simulink model "geometric_controller_with_estimator"  (R2024b)
settings: Solver=VariableStepAuto  StartTime=0.0  StopTime=t(end)  RelTol=1e-3
InitFcn:
  | %% UAV PARAMETERS
  | m = 0.5;
  | Ib = diag([0.0023 0.0023 0.00509]);
  | %% UAV PARAMETERS
  | m = 0.5;
  | Ib = diag([0.0023 0.0023 0.00509]);
  | 
  | %% SAMPLING TIME
  | Ts=0.001;
  | 
  | %% TRAJECTORY
  | 
  | % time
  | t = t_tot;
  | 
  | % initial position
  | p0x = points(1,1);
  | p0y = points(1,2);
  | p0z = - points(1,3); % ENU -> NED
  | p0 = [p0x p0y p0z];
  | 
  | % trajectory
  | csi_d=p; dot_csi_d=p_dot; ddot_csi_d=p_ddot;
  | psi_d=zeros(1,length(t)); dot_psi_d=zeros(1,length(t)); ddot_psi_d=zeros(1,length(t));
values from neighbouring files (symbols this model uses):
  K = zeros(1,r)    [filter_coeff.m]
  p = [p segments(i:i+2,:)]    [main_trajectory.m]
  p_ddot = [p_ddot segments_ddot(i:i+2,:)]    [main_trajectory.m]
  p_dot = [p_dot segments_dot(i:i+2,:)]    [main_trajectory.m]
  points = zeros(n,3)    [casual_points.m]    (also in defined_points.m = [0 0 0.2)
  r = 1    [filter_coeff.m]
  t_tot = [t_tot t_temp(i,:)]    [main_trajectory.m]
undefined symbols (not defined in the file or in its folder): ceil_dim, ceil_p, DiscIntNeverNeededParam, par_dim, par_p, supp_dim, support_1_p, support_2_p
libraries: simulink x4, robotcorelib x3, dspsigops x2, uavutilslib x1
settings Model: Creator=fabioruggiero  LastModifiedBy=ricca
settings ModelReferenceCC: EnableRefExpFcnMdlSchedulingChecks=on
settings RTWCC: GPUComputeCapability=3.5

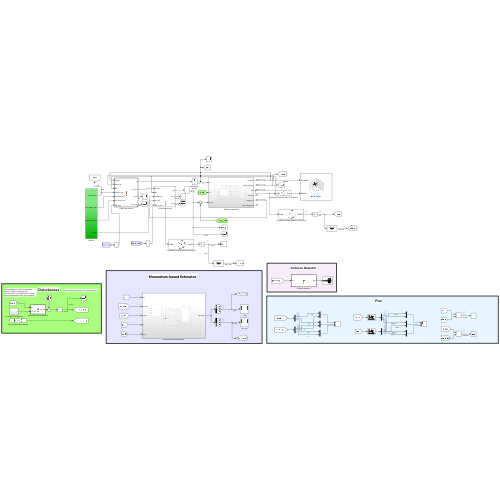
[thumbnail: Simulink's stored preview of the top-level diagram]
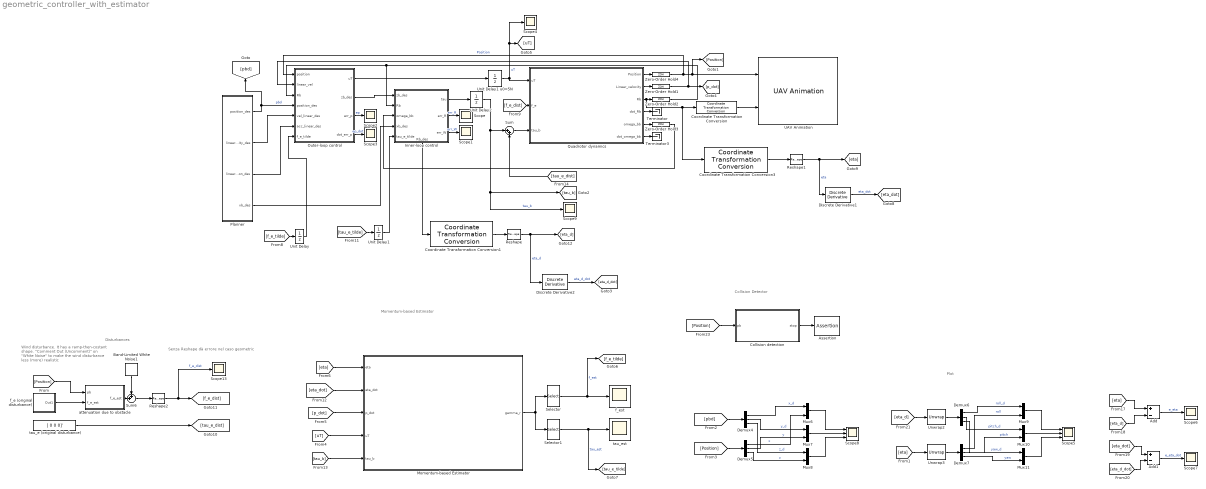
== system geometric_controller_with_estimator ==
  note: Momentum-based Estimator
  note: Collision Detector
  note: Plot
  note: Wind disturbance. It has a ramp-then-costant shape. "Comment Out (Uncomment)" on "White Noise" to make the wind disturbance less (more) realistic
  note: Senza Reshape dà errore nel caso geometric
  note: Disturbances
  Add : Sum  Inputs=+-
  Add1 : Sum  Inputs=+-
  Assertion : Assertion  AssertionFailFcn='WARNING: DRONE CRASHED!'
  Band-Limited White Noise1 : simulink/Sources/Band-Limited White Noise  Cov=[0.0001 0.0001 0]'  Ts=0.1  seed=[23341 23345 0]'  VectorParams1D=off
  Collision detection : MATLAB Function  TreatAsAtomicUnit=on
  Coordinate Transformation Conversion : robotcorelib/Coordinate Transformation Conversion  InputRepresentation=Rotation Matrix  InputEulerSequence=ZYX  ShowTrVecInputPort=on  OutputRepresentation=Quaternion  OutputEulerSequence=ZYX  ShowTrVecOutputPort=on  SimulateUsing=Interpreted execution
  Coordinate Transformation Conversion1 : robotcorelib/Coordinate Transformation Conversion  InputRepresentation=Rotation Matrix  InputEulerSequence=ZYX  ShowTrVecInputPort=on  OutputRepresentation=Euler Angles  OutputEulerSequence=XYZ  ShowTrVecOutputPort=on  SimulateUsing=Interpreted execution
  Coordinate Transformation Conversion3 : robotcorelib/Coordinate Transformation Conversion  InputRepresentation=Rotation Matrix  InputEulerSequence=ZYX  ShowTrVecInputPort=on  OutputRepresentation=Euler Angles  OutputEulerSequence=XYZ  ShowTrVecOutputPort=on  SimulateUsing=Interpreted execution
  Demux{4..7} (4 alike) : Demux  Outputs=3
  Discrete Derivative1 : simulink/Discrete/Discrete Derivative  gainval=1.0  ICPrevScaledInput=0.0  OutMin=[]  OutMax=[]  OutDataType=fixdt(1, 16)  OutScaling=2^-10  DoSatur=off
  Discrete Derivative2 : simulink/Discrete/Discrete Derivative  gainval=1.0  ICPrevScaledInput=0.0  OutMin=[]  OutMax=[]  OutDataType=fixdt(1, 16)  OutScaling=2^-10  DoSatur=off
  Inner-loop control : Subsystem  mask(Angular PID){Kr=10*eye(3), Kw=1*eye(3)}
      mask help: Kr, Kw ∈ R^(3x3) positive definite matrices
      settings: PortSchema="{\"entries\":[{\"content\":{\"sides\":[{\"content\":{\"connectorIds\":[\"In1\",\"In2\",\"In3\",\"In4\",\"In5\"]},\"type\":\"ConnectorPlacement.EquallySpacedRectSide\",\"uuid\":\"29c522b7-db36-4622-ad4a-717364e2cc35\"},{\"content\":{\"connectorIds\":[\"Out1\",\"Out2\",\"Out3\"],\"side\":\"RIGHT\"},\"type\":\"ConnectorPlacement.EquallySpacedRectSide\",\"uuid\":\"998238f4-a0c1-453d-a7e7-a110f68d17eb\"},{\"content\":{\"side\":\"TOP\"},\"type\":\"ConnectorPlacement.EquallySpacedRectSide\",\"uuid\":\"c0bfd343-7d48-415f-a23f-c8162a2dfc5d\"},{\"content\":{\"connectorIds\":[\"Out4\"],\"side\":\"BOTTOM\"},\"type\":\"ConnectorPlacement.EquallySpacedRectSide\",\"uuid\":\"eabcb074-d0a8-40eb-86b0-fc782e7c3bb4\"}]},\"type\":\"ConnectorPlacement.EquallySpacedConnector\",\"uuid\":\"fc5ab0de-d2d1-4caf-819d-5b1757328535\"}],\"packageUris\":[\"http://schema.mathworks.com/mf0/Connector/R2020b\"],\"version\":\"1.0\"}"
  Momentum-based Estimator : Subsystem
  Mux{6..11} (6 alike) : Mux  Inputs=2
  Outer-loop control : MATLAB Function  TreatAsAtomicUnit=on  mask(Linear PID){Kp=100*eye(3), Kv=100*eye(3)}
      mask help: Kp, Kv ∈ R^(3x3) positive definite matrices
  Planner : Subsystem
  Quadrotor dynamics : Subsystem
  Reshape : Reshape
  Reshape1 : Reshape
  Reshape2 : Reshape
  Scope{,1..4,6..7,9,13} (9 alike) : Scope
  Scope5 : Scope  NumInputPorts=3
  Scope8 : Scope  NumInputPorts=3
  Selector : Selector  InputPortWidth=6  IndexOptions=Index vector (dialog)  Indices=[1 2 3]  OutputSizes=1
  Selector1 : Selector  InputPortWidth=6  IndexOptions=Index vector (dialog)  Indices=[4 5 6]  OutputSizes=1
  Sum : Sum  Inputs=|++
  Sum6 : Sum  Inputs=++|
  Terminator : Terminator
  Terminator3 : Terminator
  UAV Animation : uavutilslib/UAV Animation  NumUAV=1  DynamicUAVConfig=off  UAVType=Multirotor  UAVSize=1  UAVColor=[1 0 0]  UAVTrajectoryAlpha=1  InertialZDirection=Down  RotationFormat=Quaternion  DrawMarkers=off  SampleTime=0.01
  Unit Delay : UnitDelay  SampleTime=Ts  HasFrameUpgradeWarning=on
  Unit Delay1 : UnitDelay  SampleTime=Ts  HasFrameUpgradeWarning=on
  Unit Delay1 u0=5N : UnitDelay  InitialCondition=5  SampleTime=Ts
  Unit Delay2 : UnitDelay  InitialCondition=[0 0 0]  SampleTime=Ts
  Unwrap2 : dspsigops/Unwrap  tol=pi  InputProcessing=Columns as channels (frame based)  running=off
  Unwrap3 : dspsigops/Unwrap  tol=pi  InputProcessing=Columns as channels (frame based)  running=off
  Zero-Order Hold{1..4} (4 alike) : ZeroOrderHold  SampleTime=Ts
  attenuation due to obstacle : MATLAB Function  TreatAsAtomicUnit=on
  f_e (original disturbance) : Subsystem
  f_est : Scope
  tau_e (original disturbance) : Constant  Value=[ 0 0 0]'
  tau_est : Scope
  wires:
  Unit Delay1 u0=5N/1 -> Quadrotor dynamics/1(uT), [uT], Scope4/1  "uT"
  Quadrotor dynamics/1(Position) -> Zero-Order Hold4/1
  Quadrotor dynamics/2(Linear_velocity) -> Zero-Order Hold1/1
  Quadrotor dynamics/5(omega_bb) -> Zero-Order Hold3/1
  Zero-Order Hold4/1 -> [Position], UAV Animation/1, Outer-loop control/1(position)  "Position"
  Zero-Order Hold1/1 -> [p_dot], Outer-loop control/2(linear_vel)
  Zero-Order Hold2/1 -> Outer-loop control/3(Rb), Inner-loop control/2(Rb)
  Quadrotor dynamics/4(dot_Rb) -> Terminator/1
  Planner/2(linear_velocity_des) -> Outer-loop control/5(vel_linear_des)
  Planner/3(linear_acceleration_des) -> Outer-loop control/6(acc_linear_des)
  Planner/4(xb_des) -> Inner-loop control/4(xb_des)
  Outer-loop control/3(err_p) -> Scope2/1  "ep"
  Outer-loop control/4(dot_err_p) -> Scope3/1  "ep_dot"
  Quadrotor dynamics/6(dot_omega_bb) -> Terminator3/1
  Coordinate Transformation Conversion/1 -> UAV Animation/2
  Outer-loop control/2(zb_des) -> Inner-loop control/1(zb_des)
  Zero-Order Hold3/1 -> Inner-loop control/3(omega_bb)
  Inner-loop control/1(tau) -> Unit Delay2/1
  Inner-loop control/2(err_R) -> Scope/1  "err_R"
  Inner-loop control/3(err_W) -> Scope1/1  "err_W"
  Planner/1(position_des) -> [pbd], Outer-loop control/4(position_des)  "pbd"
  Sum/1 -> Quadrotor dynamics/3(tau_b)
  Outer-loop control/1(uT) -> Unit Delay1 u0=5N/1
  Unit Delay2/1 -> Sum/1, [tau_b], Scope9/1  "tau_b"
  [tau_e_dist] -> Sum/2
  Unit Delay/1 -> Outer-loop control/7(f_e_tilde)
  Unit Delay1/1 -> Inner-loop control/5(tau_e_tilde)
  [tau_e_tilde] -> Unit Delay1/1
  [f_e_dist] -> Quadrotor dynamics/2(f_e)
  Coordinate Transformation Conversion1/1 -> Reshape/1
  Inner-loop control/4(Rb_des) -> Coordinate Transformation Conversion1/1
  Reshape/1 -> [eta_d], Discrete Derivative2/1  "eta_d"
  Discrete Derivative2/1 -> [eta_d_dot]  "eta_d_dot"
  Quadrotor dynamics/3(Rb) -> Coordinate Transformation Conversion/1, Coordinate Transformation Conversion3/1, Zero-Order Hold2/1
  Discrete Derivative1/1 -> [eta_dot]  "eta_dot"
  Coordinate Transformation Conversion3/1 -> Reshape1/1
  Reshape1/1 -> Discrete Derivative1/1, [eta]  "eta"
  [eta] -> Momentum-based Estimator/1(eta)
  [uT] -> Momentum-based Estimator/4(uT)
  [eta_dot] -> Momentum-based Estimator/2(eta_dot)
  [p_dot] -> Momentum-based Estimator/3(p_dot)
  [tau_b] -> Momentum-based Estimator/5(tau_b)
  Selector/1 -> [f_e_tilde], f_est/1  "f_est"
  Momentum-based Estimator/1(gamma_r) -> Selector/1, Selector1/1
  Selector1/1 -> [tau_e_tilde], tau_est/1  "tau_est"
  [f_e_tilde] -> Unit Delay/1
  Demux6/2 -> Mux10/1  "pitch_d"
  [eta_dot] -> Add1/1
  [eta_d_dot] -> Add1/2
  Demux4/3 -> Mux8/1  "z_d"
  Demux4/2 -> Mux7/1  "y_d"
  Demux4/1 -> Mux6/1  "x_d"
  Collision detection/1(stop) -> Assertion/1
  Mux11/1 -> Scope5/3
  Unwrap3/1 -> Demux7/1
  [Position] -> Collision detection/1(pb)
  Demux6/1 -> Mux9/1  "roll_d"
  [eta] -> Unwrap3/1
  Demux5/1 -> Mux6/2  "x"
  Demux7/2 -> Mux10/2  "pitch"
  Mux8/1 -> Scope8/3
  Demux5/3 -> Mux8/2  "z"
  Demux6/3 -> Mux11/1  "yaw_d"
  [eta] -> Add/1
  Mux6/1 -> Scope8/1
  [Position] -> Demux5/1
  Demux7/1 -> Mux9/2  "roll"
  Mux9/1 -> Scope5/1
  [eta_d] -> Unwrap2/1
  Mux10/1 -> Scope5/2
  Demux7/3 -> Mux11/2  "yaw"
  [pbd] -> Demux4/1
  [eta_d] -> Add/2
  Add1/1 -> Scope7/1  "e_eta_dot"
  Add/1 -> Scope6/1  "e_eta"
  Mux7/1 -> Scope8/2
  Unwrap2/1 -> Demux6/1
  Demux5/2 -> Mux7/2  "y"
  Sum6/1 -> Reshape2/1
  Band-Limited White Noise1/1 -> Sum6/1
  attenuation due to obstacle/1(f_e_est) -> Sum6/2
  tau_e (original disturbance)/1 -> [tau_e_dist]
  [Position] -> attenuation due to obstacle/1(pb)
  Reshape2/1 -> Scope13/1, [f_e_dist]  "f_e_dist"
  f_e (original disturbance)/1(Out1) -> attenuation due to obstacle/2("f_e_est ")

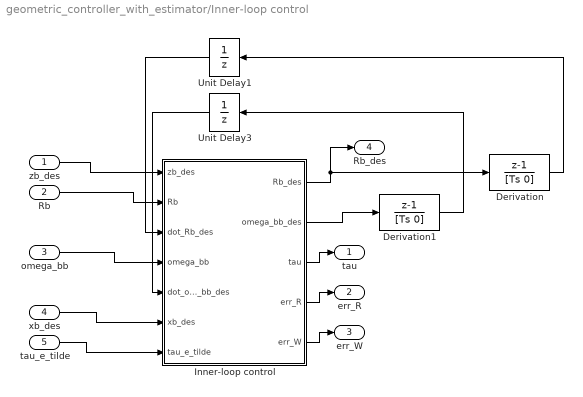
== system geometric_controller_with_estimator/Inner-loop control ==
  zb_des : Inport
  Rb : Inport  Port=2
  omega_bb : Inport  Port=3
  xb_des : Inport  Port=4
  tau_e_tilde : Inport  Port=5
  Derivation : DiscreteTransferFcn  Numerator=[1 -1]  Denominator=[Ts 0]  InitialStates=[1 0 0;0 1 0;0 0 1]  SampleTime=Ts
  Derivation1 : DiscreteTransferFcn  Numerator=[1 -1]  Denominator=[Ts 0]  InitialStates=[0 0 0]  SampleTime=Ts
  Inner-loop control : MATLAB Function  TreatAsAtomicUnit=on
  Unit Delay1 : UnitDelay  InitialCondition=eye(3)  SampleTime=Ts
  Unit Delay3 : UnitDelay  InitialCondition=[0 0 0]  SampleTime=Ts
  tau : Outport
  err_R : Outport  Port=2
  err_W : Outport  Port=3
  Rb_des : Outport  Port=4
  wires:
  xb_des/1 -> Inner-loop control/6(xb_des)
  Inner-loop control/4(err_R) -> err_R/1
  Rb/1 -> Inner-loop control/2(Rb)
  Inner-loop control/3(tau) -> tau/1
  Unit Delay1/1 -> Inner-loop control/3(dot_Rb_des)
  Derivation1/1 -> Unit Delay3/1
  Inner-loop control/5(err_W) -> err_W/1
  Unit Delay3/1 -> Inner-loop control/5(dot_omega_bb_des)
  Derivation/1 -> Unit Delay1/1
  zb_des/1 -> Inner-loop control/1(zb_des)
  omega_bb/1 -> Inner-loop control/4(omega_bb)
  Inner-loop control/2(omega_bb_des) -> Derivation1/1
  Inner-loop control/1(Rb_des) -> Derivation/1, Rb_des/1
  tau_e_tilde/1 -> Inner-loop control/7(tau_e_tilde)

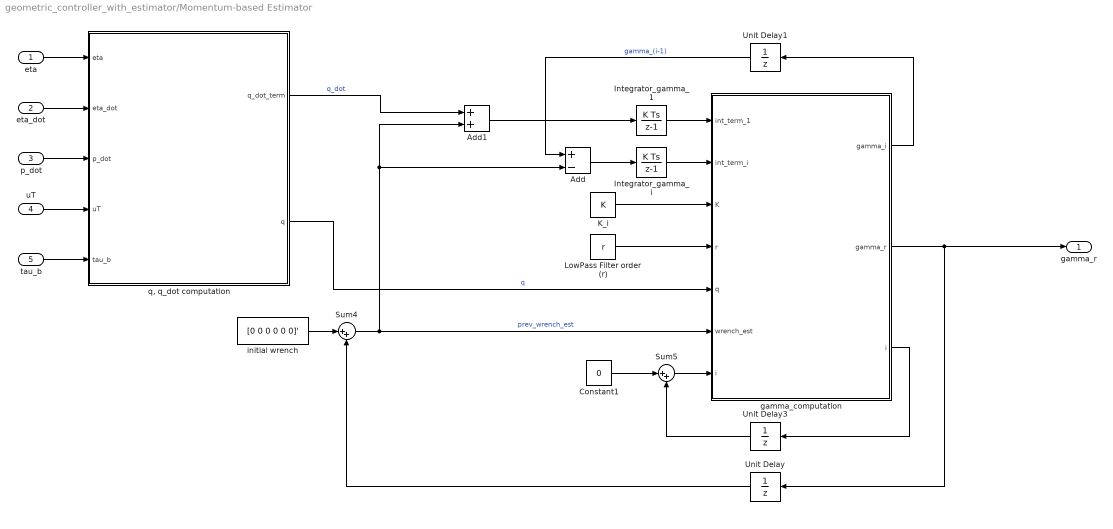
== system geometric_controller_with_estimator/Momentum-based Estimator ==
  eta : Inport
  eta_dot : Inport  Port=2
  p_dot : Inport  Port=3
  uT : Inport  Port=4
  tau_b : Inport  Port=5
  Add : Sum  Inputs=+-
  Add1 : Sum
  Constant1 : Constant  Value=0
  Integrator_gamma_1 : DiscreteIntegrator  SampleTime=Ts  ICPrevOutput=DiscIntNeverNeededParam  ICPrevScaledInput=DiscIntNeverNeededParam
  Integrator_gamma_i : DiscreteIntegrator  SampleTime=Ts  ICPrevOutput=DiscIntNeverNeededParam  ICPrevScaledInput=DiscIntNeverNeededParam
  K_i : Constant  Value=K
  LowPass Filter order (r) : Constant  Value=r
  Sum4 : Sum  Inputs=|++
  Sum5 : Sum  Inputs=|++
  Unit Delay : UnitDelay  SampleTime=Ts  HasFrameUpgradeWarning=on
  Unit Delay1 : UnitDelay  SampleTime=Ts  HasFrameUpgradeWarning=on
  Unit Delay3 : UnitDelay  SampleTime=Ts  HasFrameUpgradeWarning=on
  gamma_computation : MATLAB Function  TreatAsAtomicUnit=on
  initial wrench : Constant  Value=[0 0 0 0 0 0]'
  "q, q_dot computation" : MATLAB Function  TreatAsAtomicUnit=on
  gamma_r : Outport
  wires:
  Unit Delay/1 -> Sum4/2
  p_dot/1 -> "q, q_dot computation"/3(p_dot)
  LowPass Filter order (r)/1 -> gamma_computation/4(r)
  Sum4/1 -> gamma_computation/6(wrench_est), Add/2, Add1/2  "prev_wrench_est"
  gamma_computation/2(gamma_r) -> Unit Delay/1, gamma_r/1
  Add1/1 -> Integrator_gamma_1/1
  Add/1 -> Integrator_gamma_i/1
  Unit Delay1/1 -> Add/1  "gamma_(i-1)"
  gamma_computation/1(gamma_i) -> Unit Delay1/1
  Constant1/1 -> Sum5/1
  uT/1 -> "q, q_dot computation"/4(uT)
  "q, q_dot computation"/1(q_dot_term) -> Add1/1  "q_dot"
  K_i/1 -> gamma_computation/3(K)
  initial wrench/1 -> Sum4/1
  Integrator_gamma_1/1 -> gamma_computation/1(int_term_1)
  "q, q_dot computation"/2(q) -> gamma_computation/5(q)  "q"
  Sum5/1 -> gamma_computation/7("i ")
  Integrator_gamma_i/1 -> gamma_computation/2(int_term_i)
  gamma_computation/3(i) -> Unit Delay3/1
  Unit Delay3/1 -> Sum5/2
  eta_dot/1 -> "q, q_dot computation"/2(eta_dot)
  tau_b/1 -> "q, q_dot computation"/5(tau_b)
  eta/1 -> "q, q_dot computation"/1(eta)

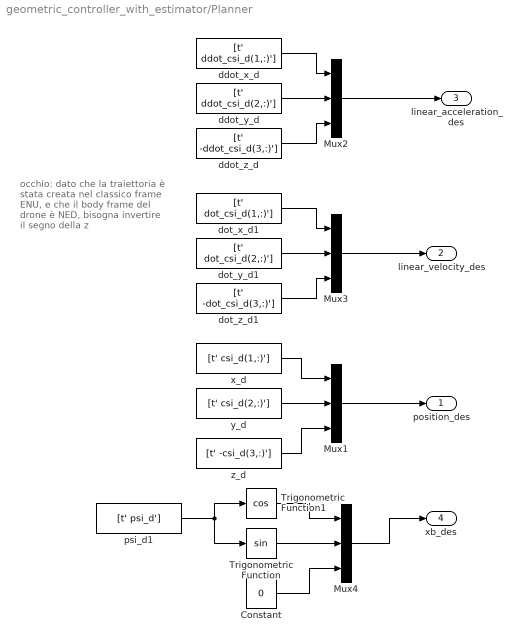
== system geometric_controller_with_estimator/Planner ==
  note: occhio: dato che la traiettoria è stata creata nel classico frame ENU, e che il body frame del drone è NED, bisogna invertire il segno della z
  Constant : Constant  Value=0
  Mux{1..4} (4 alike) : Mux  Inputs=3
  Trigonometric Function : Trigonometry
  Trigonometric Function1 : Trigonometry  Operator=cos
  ddot_x_d : FromWorkspace  VariableName=[t' ddot_csi_d(1,:)']  SampleTime=Ts
  ddot_y_d : FromWorkspace  VariableName=[t' ddot_csi_d(2,:)']  SampleTime=Ts
  ddot_z_d : FromWorkspace  VariableName=[t' -ddot_csi_d(3,:)']  SampleTime=Ts
  dot_x_d1 : FromWorkspace  VariableName=[t' dot_csi_d(1,:)']  SampleTime=Ts
  dot_y_d1 : FromWorkspace  VariableName=[t' dot_csi_d(2,:)']  SampleTime=Ts
  dot_z_d1 : FromWorkspace  VariableName=[t' -dot_csi_d(3,:)']  SampleTime=Ts
  psi_d1 : FromWorkspace  VariableName=[t' psi_d']  SampleTime=Ts
  x_d : FromWorkspace  VariableName=[t' csi_d(1,:)']  SampleTime=Ts
  y_d : FromWorkspace  VariableName=[t' csi_d(2,:)']  SampleTime=Ts
  z_d : FromWorkspace  VariableName=[t' -csi_d(3,:)']  SampleTime=Ts
  position_des : Outport
  linear_velocity_des : Outport  Port=2
  linear_acceleration_des : Outport  Port=3
  xb_des : Outport  Port=4
  wires:
  y_d/1 -> Mux1/2
  z_d/1 -> Mux1/3
  x_d/1 -> Mux1/1
  ddot_y_d/1 -> Mux2/2
  ddot_z_d/1 -> Mux2/3
  ddot_x_d/1 -> Mux2/1
  Mux2/1 -> linear_acceleration_des/1
  Mux1/1 -> position_des/1
  dot_y_d1/1 -> Mux3/2
  dot_z_d1/1 -> Mux3/3
  dot_x_d1/1 -> Mux3/1
  Mux3/1 -> linear_velocity_des/1
  Mux4/1 -> xb_des/1
  Trigonometric Function/1 -> Mux4/2
  psi_d1/1 -> Trigonometric Function/1, Trigonometric Function1/1
  Trigonometric Function1/1 -> Mux4/1
  Constant/1 -> Mux4/3

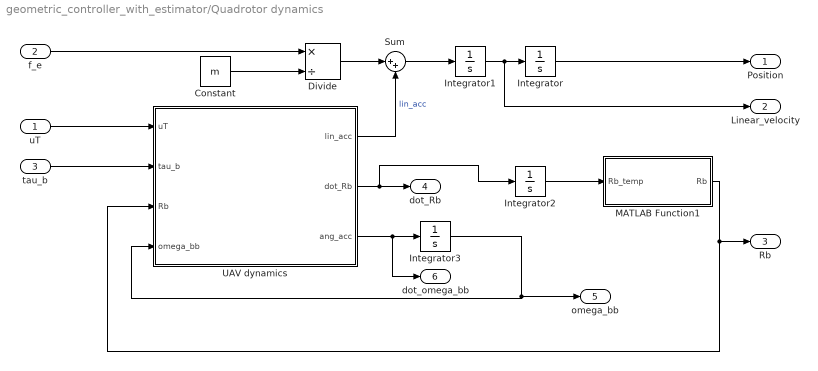
== system geometric_controller_with_estimator/Quadrotor dynamics ==
  uT : Inport
  f_e : Inport  Port=2
  tau_b : Inport  Port=3
  Constant : Constant  Value=m
  Divide : Product  Inputs=*/
  Integrator : Integrator  InitialCondition=p0
  Integrator1 : Integrator  InitialCondition=[0 0 0]
  Integrator2 : Integrator  InitialCondition=[1 0 0; 0 1 0;0 0 1]
  Integrator3 : Integrator  InitialCondition=[0 0 0]
  MATLAB Function1 : MATLAB Function  TreatAsAtomicUnit=on
  Sum : Sum  Inputs=|++
  UAV dynamics : MATLAB Function  TreatAsAtomicUnit=on
  Position : Outport
  Linear_velocity : Outport  Port=2
  Rb : Outport  Port=3
  dot_Rb : Outport  Port=4
  omega_bb : Outport  Port=5
  dot_omega_bb : Outport  Port=6
  wires:
  tau_b/1 -> UAV dynamics/2(tau_b)
  Integrator/1 -> Position/1
  UAV dynamics/3(ang_acc) -> dot_omega_bb/1, Integrator3/1
  Sum/1 -> Integrator1/1
  uT/1 -> UAV dynamics/1(uT)
  Integrator1/1 -> Linear_velocity/1, Integrator/1
  Integrator3/1 -> UAV dynamics/4(omega_bb), omega_bb/1
  UAV dynamics/2(dot_Rb) -> Integrator2/1, dot_Rb/1
  MATLAB Function1/1(Rb) -> Rb/1, UAV dynamics/3(Rb)
  Integrator2/1 -> MATLAB Function1/1(Rb_temp)
  f_e/1 -> Divide/1
  Divide/1 -> Sum/1
  Constant/1 -> Divide/2
  UAV dynamics/1(lin_acc) -> Sum/2  "lin_acc"

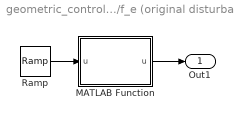
== system geometric_controller_with_estimator/f_e (original disturbance) ==
  MATLAB Function : MATLAB Function  TreatAsAtomicUnit=on
  Ramp : simulink/Sources/Ramp  slope=[ 0.1 0.1 0]'  start=5  InitialOutput=0  VectorParams1D=off
  Out1 : Outport
  wires:
  Ramp/1 -> MATLAB Function/1("u ")
  MATLAB Function/1(u) -> Out1/1

== matlab function geometric_controller_with_estimator/Momentum-based Estimator/q, q_dot computation ==
  data: eta input; eta_dot input; p_dot input; uT input; q_dot_term output; q output; tau_b input; Ib parameter; m parameter
function [q_dot_term, q] = fcn(eta, eta_dot,p_dot,uT,tau_b,Ib,m)

e_3 = [0 0 1]';
g = 9.81;
I3 = eye(3);
O3 = zeros(3);

phi = eta(1);
theta = eta(2);
psi = eta(3);

phi_dot = eta_dot(1);
theta_dot = eta_dot(2);
psi_dot = eta_dot(3);


% Q(eta)
Q = [1          0       -sin(theta);
     0      cos(phi)     cos(theta)*sin(phi);
     0     -sin(phi)     cos(theta)*cos(phi)];

% Q_dot(eta)
Q_dot = [0        0                 cos(theta)*theta_dot;
         0    -sin(phi)*phi_dot    -sin(theta)*theta_dot*sin(phi) + cos(theta)*cos(phi)*phi_dot;
         0    -cos(phi)*phi_dot    -sin(theta)*theta_dot*cos(phi) - cos(theta)*sin(phi)*phi_dot];

% C(eta,eta_dot)
C = Q'*skew(Q*eta_dot)*Ib*Q + Q'*Ib*Q_dot;

% M(eta)
M = Q'*Ib*Q;

%Rb
Rb = [cos(theta)*cos(psi) (sin(phi)*sin(theta)*cos(psi)-cos(phi)*sin(psi)) (cos(phi)*sin(theta)*cos(psi)+sin(phi)*sin(psi));
      cos(theta)*sin(psi) (sin(phi)*sin(theta)*sin(psi)+cos(phi)*cos(psi)) (cos(phi)*sin(theta)*sin(psi)-sin(phi)*cos(psi));
      -sin(theta) sin(phi)*cos(theta) cos(phi)*cos(theta)];

%%% OUTPUT
q = [m*I3 O3; O3 M]*[p_dot;eta_dot];
q_dot_term = [m*g*e_3 - uT*Rb*e_3; C'*eta_dot + Q'*tau_b];

end



function S = skew(v)
if (numel(v)~= 1)
    S= [0 -v(3) v(2);
        v(3) 0 -v(1);
        -v(2) v(1) 0];
else
    S= zeros(3);
end
end

== matlab function geometric_controller_with_estimator/attenuation due to obstacle ==
  data: pb input; f_e_est input; f_e_est output; ceil_dim parameter; ceil_p parameter; supp_dim parameter
function f_e_est = fcn(pb,f_e_est,ceil_dim, ceil_p, supp_dim)

% quadrotor coordinates
x = pb(1);
y = pb(2);
z = pb(3); % ricordare che ha segno negativo (NED frame)

% OCCHIO: ricordare che nella configurazione NED le z sono NEGATIVE!!!
% Quindi devi ragionare al contrario per le condizioni di passaggio
% nell'ostacolo

% CONDIZIONE PASSAGGIO ALL'INTERNO DEL PRIMO OSTACOLO
if       x >= ceil_p(1) - ceil_dim(1)/2                  &&   x <= ceil_p(1) + ceil_dim(1)/2                    && ...
         y >= ceil_p(2) - (ceil_dim(2)/2 - supp_dim(2))  &&   y <= ceil_p(2) + (ceil_dim(2)/2 - supp_dim(2))    && ...
         z >= -supp_dim(3)                               &&   z <= 0
    
    if f_e_est(2) >= 0.1            % Se c'è vento moderato lungo l'asse y ...
        f_e_est(2) = f_e_est(2)/2;  % ...dimezzo la sua intensità lungo tale asse, perché impatta contro il supporto dell'ostacolo.
    else                            % Se il vento è di bassa intensità lungo l'asse y ...
        f_e_est(2) = 0;             % l'impatto con il support blocca completamente il vento lungo tale asse. 
    end
end

end

== matlab function geometric_controller_with_estimator/Collision detection ==
  data: pb input; stop output; ceil_p parameter; par_p parameter; ceil_dim parameter; par_dim parameter; supp_dim parameter; support_1_p parameter; support_2_p parameter
function stop =  f(pb, ceil_p, par_p, ceil_dim, par_dim, supp_dim, support_1_p, support_2_p)

% OCCHIO: le dimensioni degli ostacoli e le dimensioni x e y della posizione
% del drone sono positive. La dimensione z del drone NO: sono negative 
% (NED frame)! Attento nelle formule e nelle condizioni dei costrutti 
% if/else

% Dovrò tenere in conto anche della mesh del drone:

% ** Maximum width with propeller = 0.57 m -> maximum radius with propeller = 0.285 m
r = 0.285;

% ** Height = 0.1 m -> distance "center of mass - upper/lower" tip = 0.05 m
h = 0.05;

%% INITIALIZATION
stop = 1; % if no collision -> stop = 1

x = pb(1);
y = pb(2);
z = pb(3); % it is a negative value because of the NED configuration


%% COLLISION DETECTION
% if there is a collision -> stop = 0 

% Collision with the ground
if              z >= 0 - h
    stop = 0;

% Collision with the ceiling
elseif          x >= ceil_p(1) - ceil_dim(1)/2 - r                  &&   x <= ceil_p(1) + ceil_dim(1)/2 + r               && ... % le condizioni sull'asse x sono state fatte rispetto alla posizione del centro e alle dimensioni rispetto a x del soffitto
                y >= ceil_p(2) - ceil_dim(2)/2 - r                  &&   y <= ceil_p(2) + ceil_dim(2)/2 + r               && ... % le condizioni sull'asse y sono state fatte rispetto alla posizione del centro e alle dimensioni rispetto a y del soffitto
                z <= -supp_dim(3) + h                               &&   z >= -(supp_dim(3) + ceil_dim(3)) - h                   % le condizioni sull'asse z sono state fatte rispetto all'altezza dei sostegni (supposti uguali) + lo spessore del soffitto (dimensione in z)

    stop = 0; % STOP VALUE

% Collision with the 1st ceiling support
elseif          x >= support_1_p(1) - supp_dim(1)/2 - r             &&   x <= support_1_p(1) + supp_dim(1)/2 + r          && ... % le condizioni sull'asse x sono state fatte rispetto alla posizione del centro e alle dimensioni rispetto a x del primo supporto (con supporti supposti uguali)
                y >= support_1_p(2) - supp_dim(2)/2 - r             &&   y <= support_1_p(2) + supp_dim(2)/2 + r          && ... % le condizioni sull'asse y sono state fatte rispetto alla posizione del centro e alle dimensioni rispetto a y del primo supporto (con supporti supposti uguali)
                z <= 0 + h                                          &&   z >= -supp_dim(3) - h                                   % le condizioni sull'asse z sono state fatte rispetto all'altezza dei sostegni (supposti uguali) + lo spessore del soffitto (dimensione in z)

    stop = 0; % STOP VALUE

% Collision with the 2nd ceiling support
elseif          x >= support_2_p(1) - supp_dim(1)/2 - r             &&   x <= support_2_p(1) + supp_dim(1)/2 + r          && ... % le condizioni sull'asse x sono state fatte rispetto alla posizione del centro e alle dimensioni rispetto a x del secondo supporto (con supporti supposti uguali)
                y >= support_2_p(2) - supp_dim(2)/2 - r             &&   y <= support_2_p(2) + supp_dim(2)/2 + r          && ... % le condizioni sull'asse y sono state fatte rispetto alla posizione del centro e alle dimensioni rispetto a y del secondo supporto (con supporti supposti uguali)
                z <= 0 + h                                          &&   z >= -supp_dim(3) - h                                   % le condizioni sull'asse z sono state fatte rispetto all'altezza dei sostegni (supposti uguali) + lo spessore del soffitto (dimensione in z)

    stop = 0; % STOP VALUE

% Collision with the  parallelepiped
elseif          x >= par_p(1) - par_dim(1)/2 - r                    &&   x <= par_p(1) + par_dim(1)/2 + r                  && ... % le condizioni sull'asse x sono state fatte rispetto alla posizione del centro e alle dimensioni rispetto a x della colonna (parallelepipedo)
                y >= par_p(2) - par_dim(2)/2 - r                    &&   y <= par_p(2) + par_dim(2)/2 + r                  && ... % le condizioni sull'asse y sono state fatte rispetto alla posizione del centro e alle dimensioni rispetto a y della colonna (parallelepipedo)
                z <= 0 + h                                          &&   z >= -par_dim(3) - h                                     % le condizioni sull'asse z sono state fatte rispetto all'altezza della colonna partendo dal pavimento (dimensione in z)

    stop = 0; % STOP VALUE

end

end

== matlab function geometric_controller_with_estimator/f_e (original disturbance)/MATLAB Function ==
  data: u input; u output
function u = fcn(u)
if u >= [0.1 0.1 0]'
    u = [0.1 0.1 0]';
end

== matlab function geometric_controller_with_estimator/Quadrotor dynamics/UAV dynamics ==
  data: uT input size=1; tau_b input size=3; lin_acc output size=3; Rb input size=[3,3]; omega_bb input size=3; dot_Rb output size=[3,3]; ang_acc output size=3; m parameter size=1; Ib parameter size=[3,3]
function [lin_acc, dot_Rb, ang_acc] = fcn(uT,tau_b,Rb,omega_bb,m, Ib)

lin_acc = 9.81*[0 0 1]'-(uT/m)*Rb*[0 0 1]';
dot_Rb = Rb*skew(omega_bb);
ang_acc = inv(Ib)*(-skew(omega_bb)*Ib*omega_bb + tau_b);

end

function S = skew(v)
if(numel(v)~= 1)
S= [0 -v(3) v(2); 
    v(3) 0 -v(1);
    -v(2) v(1) 0];
else
S= zeros(3);
end
end

== matlab function geometric_controller_with_estimator/Outer-loop control ==
  data: position input size=3; uT output size=1; linear_vel input size=3; Rb input size=[3,3]; zb_des output size=3; m parameter size=1; position_des input size=3; vel_linear_des input size=3; acc_linear_des input size=3; err_p output size=3; dot_err_p output size=3; f_e_tilde input; Kp parameter; Kv parameter
function [uT, zb_des, err_p, dot_err_p] = fcn(position, linear_vel, Rb, m, ...
    position_des, vel_linear_des, acc_linear_des, f_e_tilde,Kp, Kv)

%% WRITE HERE THE OUTER-LOOP CONTROL
% position: linear position measure
% linear_vel: linear velocity measure
% Rb: current rotation matrix
% mass: mass of the UAV
% positon_des: desired linear position from the planner
% vel_linear_des: desired linear velocity from the planner
% acc_linear_des: desired linear acceleration from the planner
% ---
% uT: commanded total thrust
% zb_des: desired z-axis of the body frame
% err_p: position error
% dot_err_p: time derivative of the positon error

e3 = [0 0 1]';
err_p = position - position_des;
dot_err_p = linear_vel - vel_linear_des;


% acceleration handling. Solitamente la costante di comparazione è 
% "m*9.81". Infatti non voglio che il drone, soggetto alla forza di
% gravità, acceleri verso il basso con accelerazione maggiore di 
% g = -9.81 m/s^2.
handler = - m*9.81*e3 + m*acc_linear_des;
if handler(3) >= m*9.81
    handler(3) = m*9.8;
elseif handler(3) <= - m*9.81
    handler(3) = - m*9.8;
end


% control law & zb_des
uT = - (- Kp*err_p - Kv*dot_err_p + handler - f_e_tilde)'*Rb*e3;
zb_des = - (- Kp*err_p - Kv*dot_err_p + handler - f_e_tilde)/norm(- Kp*err_p - Kv*dot_err_p - m*9.81*e3 + m*acc_linear_des - f_e_tilde);

== matlab function geometric_controller_with_estimator/Inner-loop control/Inner-loop control ==
  data: Rb_des output size=[3,3]; omega_bb_des output size=3; tau output size=3; zb_des input size=3; Rb input size=[3,3]; dot_Rb_des input size=[3,3]; omega_bb input size=3; dot_omega_bb_des input size=3; xb_des input size=3; Ib parameter size=[3,3]; err_R output size=3; err_W output size=3; tau_e_tilde input; Kr parameter; Kw parameter
function [Rb_des,omega_bb_des,tau,err_R,err_W] = fcn(zb_des,Rb,dot_Rb_des,omega_bb,dot_omega_bb_des,xb_des,Ib, tau_e_tilde,Kr, Kw)

%% WRITE HERE THE INNER-LOOP CONTROL
% zb_des: desired z-axis of the body frame
% Rb: current rotation matrix
% dot_Rb_des: time-derivative of the desired rotation matrix
% omega_bb: current angular velocity expressed in the body frame
% dot_omega_bb_des: desired angular acceleration expressed in the body
% frame
% xb_des: desired x-axis of the body frame form the planner
% Ib: inertia matrix of the UAV with respect to the body frame
% ---
% Rb_des: desired rotation matrix
% omega_bb_des: desired angular velocity expressed in the body frame (given
% below as a hint)
% tau: commanded control torque
% err_R: rotational error in SO(3)
% err_W: angular velocity error in SO(3)

yb_des = (skew(zb_des)*xb_des)/norm(skew(zb_des)*xb_des);
xb_des = skew(yb_des)*zb_des;
Rb_des = [xb_des yb_des zb_des];

omega_bb_des = wedge(Rb_des'*dot_Rb_des);

err_R = 1/2*wedge(Rb_des'*Rb - Rb'*Rb_des);
err_W = omega_bb - Rb'*Rb_des*omega_bb_des;


tau = - Kr*err_R - Kw*err_W + skew(omega_bb)*Ib*omega_bb - Ib*(skew(omega_bb)*Rb'*Rb_des*omega_bb_des - Rb'*Rb_des*dot_omega_bb_des) - tau_e_tilde;

end

function S = skew(v)
if(numel(v)~= 1)
S= [0 -v(3) v(2); 
    v(3) 0 -v(1);
    -v(2) v(1) 0];
else
S= zeros(3);
end
end

function v = wedge(S)
v1 = S(3,2);
v2 = S(1,3);
v3 = S(2,1);
v = [v1 v2 v3]';
end

== matlab function geometric_controller_with_estimator/Quadrotor dynamics/MATLAB Function1 ==
  data: Rb_temp input; Rb output
function Rb = fcn(Rb_temp)
    [U,S,V] = svd(Rb_temp);
    sigma = det(U*V');
    S_ = diag([1 1 sigma]);

    Rb = U*S_*V';
end

== matlab function geometric_controller_with_estimator/Momentum-based Estimator/gamma_computation ==
  data: int_term_1 input; int_term_i input; K input; r input; q input; wrench_est input; gamma_i output; gamma_r output; i input; i output
function [gamma_i,gamma_r, i] = fcn(int_term_1, int_term_i,K,r,q, wrench_est, i)
gamma_r = wrench_est;
gamma_i = zeros(6,1);

if r == 1 % quando è di ordine 1
    gamma_i = K(1)*eye(6)*(q-int_term_1); % infatti i coefficienti riguardano il i-esimo filtro Gi(s) con i = 1,...,6. Quindi abbiamo 6 coefficienti per i 6 filtri
    gamma_r = gamma_i;
else % quando l'ordine è maggiore di 1
    if i == 0
        i = i+1;
        gamma_i = K(1)*eye(6)*(q-int_term_1);
    else
        i = i+1;
        gamma_i = K(i)*eye(6)*int_term_i;
        if i == r
            gamma_r = gamma_i;
            i = 0;
        end
    end
end

end
